simulink model "IO301interruptsynchsubsystem"  (Simulink 7.5)
settings: Solver=FixedStepDiscrete  StartTime=0.0  StopTime=inf  RelTol=1e-3
PreLoadFcn:
  | fpga_freq = 33e6;
  | Ts = 0.001;
  | Tpwm = 100e-6;
undefined symbols (not defined in the file): ATI, R5, RP
libraries: xpclib x3, speedgoatlib_IO301 x3, simulink x1
settings Model: Creator=dkuratli  LastModifiedBy=lab3  BufferReuse=off
settings OptimizationCC: BlockReduction=off  OptimizeBlockIOStorage=off  BufferReuse=off  ExpressionFolding=off  ExpressionDepthLimit=128  LocalBlockOutputs=off
settings DebuggingCC: UnderspecifiedInitializationDetection=Simplified  FcnCallInpInsideContextMsg=Enable All  StateNameClashWarn=none
settings HardwareCC: ProdIntDivRoundTo=Zero  ProdEndianess=LittleEndian  ProdHWDeviceType=Generic->32-bit x86 compatible
settings RTWCC: SystemTargetFile=xpctarget.tlc  TemplateMakefile=xpc_default_tmf  Description=Simulink Real-Time  RTWVerbose=off  ProcessScript=xpctarget_make_rtw_hook  RTWCompilerOptimization=On
settings CodeAppCC: CustomSymbolStrType=$N$R$M_T
settings xpcTargetCC: TargetFcnLib=ansi_tfl_table_tmw.mat  TargetFunctionLibrary=ANSI_C  ParMdlRefBuildCompliant=on  ConcurrentExecutionCompliant=on  CombineSignalStateStructs=off  GRTInterface=on  GenerateAllocFcn=off  xPCTaskExecutionProfile=off  xPCRL32EventNumber=5000  xPCLoadParamSetFile=off  xPCConcurrentTasks=off  xPCEnableSFAnimation=off

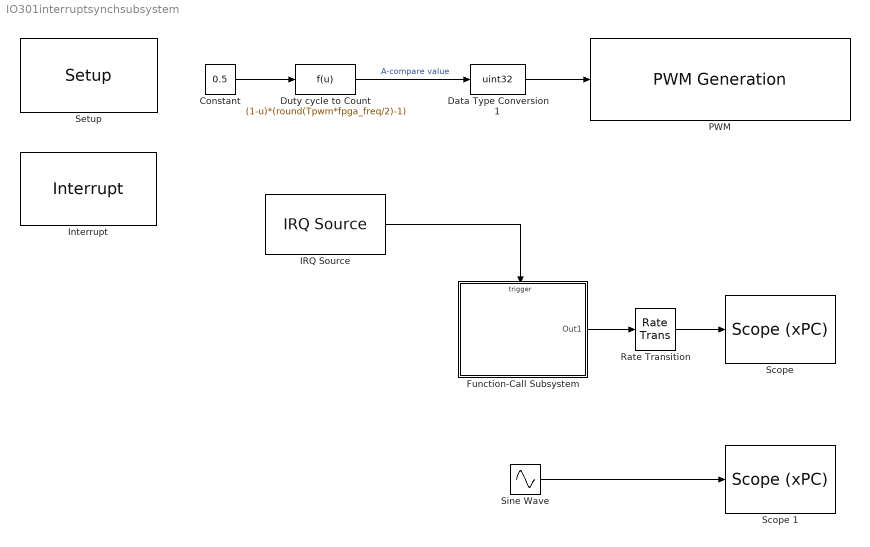
== system IO301interruptsynchsubsystem ==
  Constant : Constant  Value=0.5  SampleTime=Ts
  Data Type Conversion1 : DataTypeConversion  OutDataTypeStr=uint32  OutDataTypeMode=uint32
  Duty cycle to Count : Fcn  Expr=(1-u)*(round(Tpwm*fpga_freq/2)-1)
  Function-Call Subsystem : Subsystem  TreatAsAtomicUnit=on
  "IRQ Source " : xpclib/Asynchronous Event/IRQ Source  irqNo=Auto (PCI only)  preempt=10  b_type=ATI-RP-R5  slot=-1
  Interrupt : speedgoatlib_IO301/Interrupt/Interrupt  id=1  debounce=0  delay=0  polarity=0  pciSlot=-1  ts=-1
  PWM : speedgoatlib_IO301/PWM Generation/PWM Generation  channel=[1]  group=Module setup  id=1  ts=-1  pciSlot=-1  initStart=[1]  toggleAStart=[0]  toggleAStop=[0]  toggleBStart=[1]  toggleBStop=[0]  showStart=off  showAStart=off  showAStop=off  showBStart=off  showBStop=off  initA=[1]  initB=[1]  initC=[round(fpga_freq*Tpwm/2)-1]  showA=on  showB=off  showC=off  initActionA=[0,0,2,1]'  initActionB=[0,0,2,1]'  showActionA=off  showActionB=off  triggerSource=[1]  triggerPulseLength=32  protection=[0]
  Rate Transition : RateTransition  Deterministic=off
  "Scope " : xpclib/Misc./Scope (xPC)   scopeno=1  scopetype=Target  autostart=on  viewmode=Numerical  formatstr='%15.6f'  grid=on  ylimits=[0,0]  nosamples=3  noprepostsamples=0  interleave=1  triggermode=FreeRun  triggersignal=1  trigsignalfromport=off  triggerlevel=0.0  triggerslope=Either  triggerscope=1  triggersample=0  filename=data.dat  mode=Lazy  writesize=512  autorestart=off  dynamicfilemode=off  maxwritefilesize=512*1024^2
  Scope 1 : xpclib/Misc./Scope (xPC)   scopeno=2  scopetype=Target  autostart=on  viewmode=Graphical redraw  formatstr='%15.6f'  grid=on  ylimits=[0,0]  nosamples=250  noprepostsamples=0  interleave=1  triggermode=FreeRun  triggersignal=1  trigsignalfromport=off  triggerlevel=0.0  triggerslope=Either  triggerscope=1  triggersample=0  filename=data.dat  mode=Lazy  writesize=512  autorestart=off  dynamicfilemode=off  maxwritefilesize=512*1024^2
  Setup : speedgoatlib_IO301/Setup/Setup  group=Module setup  id=1  fpga1=speedgoat_IO301_default  pciSlot=-1  lowerDirection=[1, 1, 1, 1, 1, 0, 0, 0, 0, 0, 0, 0, 1, 1, 1, 1]  lowerReset=[1]  lowerValue=[0]  upperDirection=[1, 1, 1, 1, 1, 1, 1, 1, 0, 0, 0, 0, 0, 0, 0, 0]  upperReset=[1]  upperValue=[0]
  Sine Wave : Sin  Amplitude=[1, 2, 3]  Frequency=2*pi*10  SampleTime=Ts
  wires:
  Duty cycle to Count/1 -> Data Type Conversion1/1  "A-compare value"
  Data Type Conversion1/1 -> PWM/1
  Constant/1 -> Duty cycle to Count/1
  "IRQ Source "/1 -> Function-Call Subsystem/Trigger
  Function-Call Subsystem/1(Out1) -> Rate Transition/1
  Sine Wave/1 -> Scope 1/1
  Rate Transition/1 -> "Scope "/1

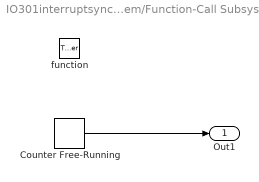
== system IO301interruptsynchsubsystem/Function-Call Subsystem ==
  function : TriggerPort  TriggerType=function-call
  Counter Free-Running : simulink/Sources/Counter Free-Running  NumBits=32  tsamp=-1
  Out1 : Outport
  wires:
  Counter Free-Running/1 -> Out1/1
